simulink model "Simple_Joystick_SIM"  (R2025b)
settings: Solver=FixedStepAuto  StartTime=0.0  StopTime=tspan  FixedStep=dt_sim  RelTol=1e-3
undefined symbols (not defined in the file): const_joy, const_voltage, dt_control
settings Model: Creator=vulcangrip  LastModifiedBy=koryh
settings OptimizationCC: DefaultParameterBehavior=Inlined  EnhancedBackFolding=on  PassReuseOutputArgsAs=Individual arguments  ZeroExternalMemoryAtStartup=off  ZeroInternalMemoryAtStartup=off  MaxStackSize=64  OptimizeBlockOrder=speed  DifferentSizesBufferReuse=on  OptimizationCustomize=off  EfficientTunableParamExpr=on
settings DebuggingCC: ParameterTunabilityLossMsg=error
settings HardwareCC: ProdBitPerLong=64.0  ProdHWDeviceType=Intel->x86-64 (Linux 64)
settings SFSimCC: MATLABDynamicMemAlloc=off  SimTargetLang=C++  SimDLTargetLibrary=mkl-dnn
settings RTWCC: SystemTargetFile=ert.tlc  HardwareBoard=Robot Operating System 2 (ROS 2)  TLCOptions="-aInlineSetEventsForThisBaseRateFcn=TLC_FALSE -aSuppressMultiTaskScheduler=TLC_FALSE  -aRateBasedStepFcn=0"  GenCodeOnly=on  TemplateMakefile=ert_default_tmf  Toolchain=Colcon Tools  TargetLang=C++  CheckMdlBeforeBuild=Warning  Description=Embedded Coder
settings CodeAppCC: ForceParamTrailComments=on  IgnoreCustomStorageClasses=off  OperatorAnnotations=on  SimulinkDataObjDesc=on  SFDataObjDesc=on  InsertBlockDesc=on
settings ERTTargetCC: ExtModeTransport=2.0  ExtModeStaticAlloc=on  ExtModeAutomaticAllocSize=off  ExtModeMexFile=ext_xcp  ExtModeIntrfLevel=Level2 - Open  RootIOFormat=Structure reference  TargetLangStandard=C++11 (ISO)  CodeInterfacePackaging=C++ class  SubcomponentCodeInterfacePackaging=C++ class

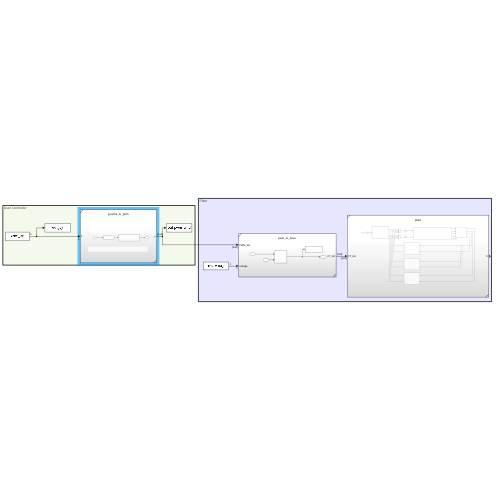
[thumbnail: Simulink's stored preview of the top-level diagram]
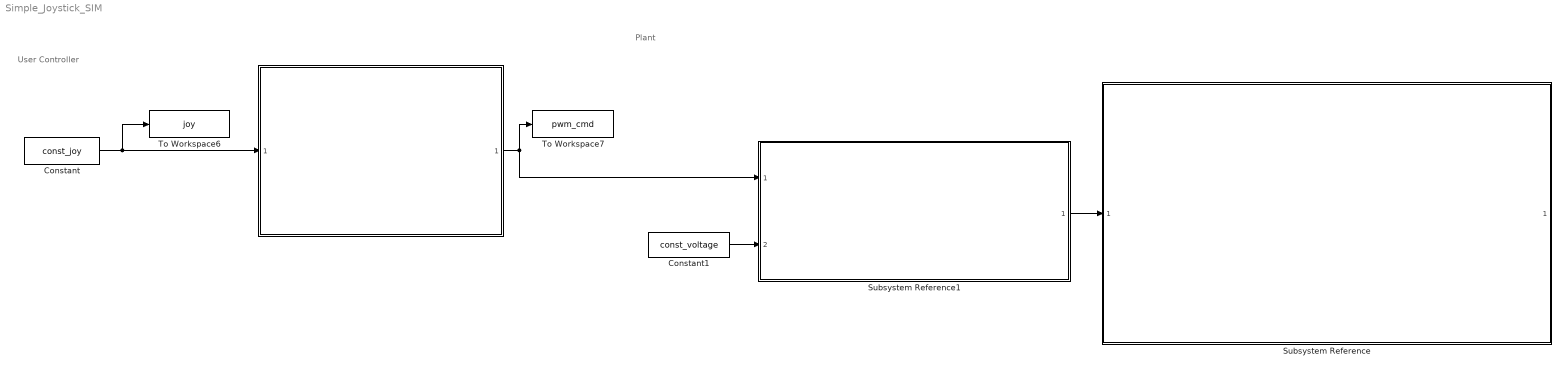
== system Simple_Joystick_SIM ==
  note: Plant
  note: User Controller
  " " : Subsystem  ReferencedSubsystem=joystick_to_pwm
  Constant : Constant  Value=const_joy
  Constant1 : Constant  Value=const_voltage
  Subsystem Reference : Subsystem  ReferencedSubsystem=plant
  Subsystem Reference1 : Subsystem  ReferencedSubsystem=pwm_to_force
  To Workspace6 : ToWorkspace  VariableName=joy  SaveFormat=Timeseries  SampleTime=dt_control
  To Workspace7 : ToWorkspace  VariableName=pwm_cmd  SaveFormat=Timeseries  SampleTime=dt_control
  wires:
  " "/1 -> To Workspace7/1, Subsystem Reference1/1
  Constant/1 -> " "/1, To Workspace6/1
  Subsystem Reference1/1 -> Subsystem Reference/1
  Constant1/1 -> Subsystem Reference1/2
